simulink model "IIR_Transposed_Direct_Form_II"  (R2012b)
settings: Solver=ode45  StartTime=0.0  StopTime=10.0  RelTol=1e-3
settings Model: Creator=Ahmad  LastModifiedBy=Ahmad

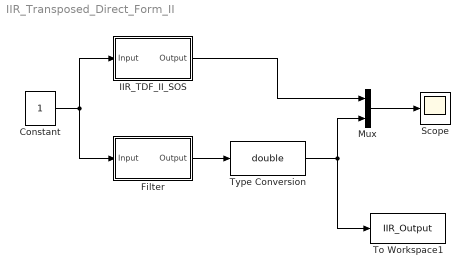
== system IIR_Transposed_Direct_Form_II ==
  Constant : Constant  VectorParams1D=off  OutDataTypeStr=double  SampleTime=1/50e6
  Filter : Subsystem  Tag=FilterWizardSubSystem
      settings: ErrorFcn=dspFilterRealizedInBasicElemsAlgLoopErrFcnCallback
  IIR_TDF_II_SOS : Subsystem  Tag=FilterWizardSubSystem
      settings: ErrorFcn=dspFilterRealizedInBasicElemsAlgLoopErrFcnCallback
  Mux : Mux  Inputs=2
  Scope : Scope
      settings: YMin=0.1  YMax=0.85
  To Workspace1 : ToWorkspace  VariableName=IIR_Output  SampleTime=-1  SaveFormat=Timeseries
  Type Conversion : DataTypeConversion  OutDataTypeStr=double
  wires:
  Constant/1 -> Filter/1(Input), IIR_TDF_II_SOS/1(Input)
  Filter/1(Output) -> Type Conversion/1
  Mux/1 -> Scope/1
  IIR_TDF_II_SOS/1(Output) -> Mux/1
  Type Conversion/1 -> To Workspace1/1, Mux/2

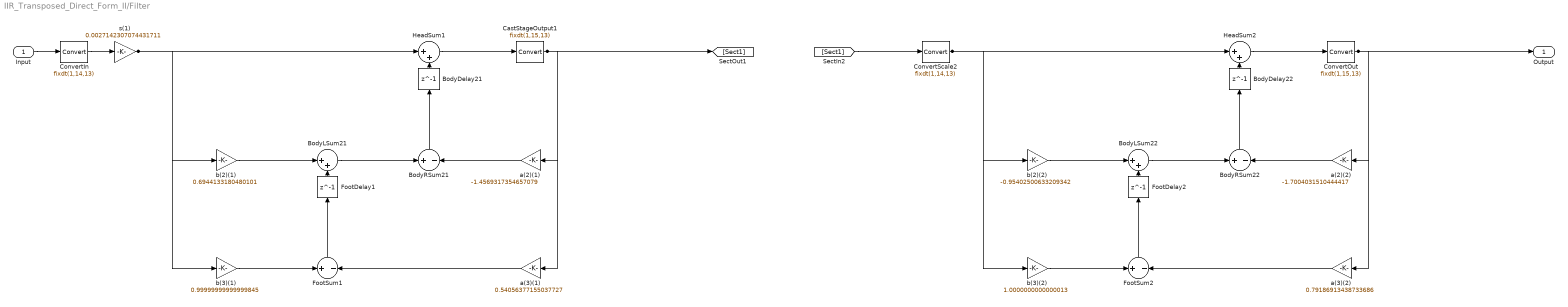
== system IIR_Transposed_Direct_Form_II/Filter ==
  Input : Inport
  BodyDelay21 : Delay  DelayLength=1  InitialCondition=0
  BodyDelay22 : Delay  DelayLength=1  InitialCondition=0
  BodyLSum21 : Sum  Inputs=|++  AccumDataTypeStr=fixdt(1,28,24)  OutDataTypeStr=fixdt(1,28,24)
  BodyLSum22 : Sum  Inputs=|++  AccumDataTypeStr=fixdt(1,28,24)  OutDataTypeStr=fixdt(1,28,24)
  BodyRSum21 : Sum  Inputs=+|-  AccumDataTypeStr=fixdt(1,28,24)  OutDataTypeStr=fixdt(1,28,24)
  BodyRSum22 : Sum  Inputs=+|-  AccumDataTypeStr=fixdt(1,28,24)  OutDataTypeStr=fixdt(1,28,24)
  CastStageOutput1 : DataTypeConversion  OutDataTypeStr=fixdt(1,15,13)
  ConvertIn : DataTypeConversion  OutDataTypeStr=fixdt(1,14,13)  RndMeth=Nearest  SaturateOnIntegerOverflow=on
  ConvertOut : DataTypeConversion  OutDataTypeStr=fixdt(1,15,13)
  ConvertScale2 : DataTypeConversion  OutDataTypeStr=fixdt(1,14,13)
  FootDelay1 : Delay  DelayLength=1  InitialCondition=0
  FootDelay2 : Delay  DelayLength=1  InitialCondition=0
  FootSum1 : Sum  Inputs=+|-  AccumDataTypeStr=fixdt(1,28,24)  OutDataTypeStr=fixdt(1,28,24)
  FootSum2 : Sum  Inputs=+|-  AccumDataTypeStr=fixdt(1,28,24)  OutDataTypeStr=fixdt(1,28,24)
  HeadSum1 : Sum  Inputs=|++  AccumDataTypeStr=fixdt(1,28,24)  OutDataTypeStr=fixdt(1,28,24)
  HeadSum2 : Sum  Inputs=|++  AccumDataTypeStr=fixdt(1,28,24)  OutDataTypeStr=fixdt(1,28,24)
  a(2)(1) : Gain  Gain=-1.4569317354657079  ParamDataTypeStr=fixdt(1,13,11)  OutDataTypeStr=fixdt(1,28,24)
  a(2)(2) : Gain  Gain=-1.7004031510444417  ParamDataTypeStr=fixdt(1,13,11)  OutDataTypeStr=fixdt(1,28,24)
  a(3)(1) : Gain  Gain=0.54056377155037727  ParamDataTypeStr=fixdt(1,13,11)  OutDataTypeStr=fixdt(1,28,24)
  a(3)(2) : Gain  Gain=0.79186913438733686  ParamDataTypeStr=fixdt(1,13,11)  OutDataTypeStr=fixdt(1,28,24)
  b(2)(1) : Gain  Gain=0.6944133180480101  ParamDataTypeStr=fixdt(1,13,11)  OutDataTypeStr=fixdt(1,28,24)
  b(2)(2) : Gain  Gain=-0.95402500633209342  ParamDataTypeStr=fixdt(1,13,11)  OutDataTypeStr=fixdt(1,28,24)
  b(3)(1) : Gain  Gain=0.99999999999999845  ParamDataTypeStr=fixdt(1,13,11)  OutDataTypeStr=fixdt(1,28,24)
  b(3)(2) : Gain  Gain=1.0000000000000013  ParamDataTypeStr=fixdt(1,13,11)  OutDataTypeStr=fixdt(1,28,24)
  s(1) : Gain  Gain=0.0027142307074431711  ParamDataTypeStr=fixdt(1,13,12)  OutDataTypeStr=fixdt(1,14,13)
  Output : Outport
  wires:
  Input/1 -> ConvertIn/1
  s(1)/1 -> HeadSum1/1, b(2)(1)/1, b(3)(1)/1
  HeadSum1/1 -> CastStageOutput1/1
  CastStageOutput1/1 -> [Sect1], a(2)(1)/1, a(3)(1)/1
  b(2)(1)/1 -> BodyLSum21/1
  BodyLSum21/1 -> BodyRSum21/1
  BodyRSum21/1 -> BodyDelay21/1
  a(2)(1)/1 -> BodyRSum21/2
  BodyDelay21/1 -> HeadSum1/2
  b(3)(1)/1 -> FootSum1/1
  FootSum1/1 -> FootDelay1/1
  a(3)(1)/1 -> FootSum1/2
  FootDelay1/1 -> BodyLSum21/2
  ConvertIn/1 -> s(1)/1
  [Sect1] -> ConvertScale2/1
  ConvertScale2/1 -> HeadSum2/1, b(2)(2)/1, b(3)(2)/1
  HeadSum2/1 -> ConvertOut/1
  ConvertOut/1 -> Output/1, a(2)(2)/1, a(3)(2)/1
  b(2)(2)/1 -> BodyLSum22/1
  BodyLSum22/1 -> BodyRSum22/1
  BodyRSum22/1 -> BodyDelay22/1
  a(2)(2)/1 -> BodyRSum22/2
  BodyDelay22/1 -> HeadSum2/2
  b(3)(2)/1 -> FootSum2/1
  FootSum2/1 -> FootDelay2/1
  a(3)(2)/1 -> FootSum2/2
  FootDelay2/1 -> BodyLSum22/2

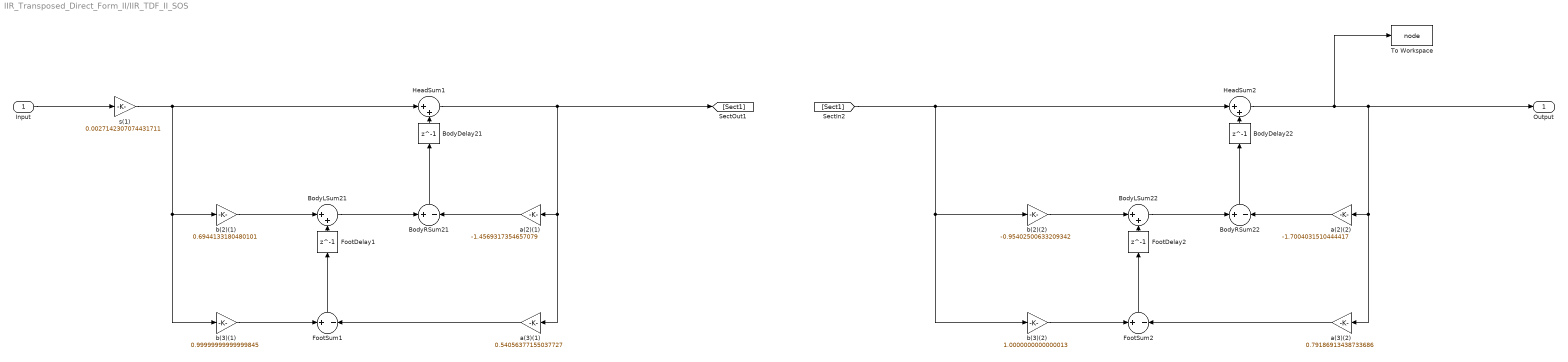
== system IIR_Transposed_Direct_Form_II/IIR_TDF_II_SOS ==
  Input : Inport
  BodyDelay21 : Delay  DelayLength=1  InitialCondition=0
  BodyDelay22 : Delay  DelayLength=1  InitialCondition=0
  BodyLSum21 : Sum  Inputs=|++  RndMeth=Nearest  SaturateOnIntegerOverflow=on  OutDataTypeStr=Inherit: Same as first input
  BodyLSum22 : Sum  Inputs=|++  RndMeth=Nearest  SaturateOnIntegerOverflow=on  OutDataTypeStr=Inherit: Same as first input
  BodyRSum21 : Sum  Inputs=+|-  RndMeth=Nearest  SaturateOnIntegerOverflow=on  OutDataTypeStr=Inherit: Same as first input
  BodyRSum22 : Sum  Inputs=+|-  RndMeth=Nearest  SaturateOnIntegerOverflow=on  OutDataTypeStr=Inherit: Same as first input
  FootDelay1 : Delay  DelayLength=1  InitialCondition=0
  FootDelay2 : Delay  DelayLength=1  InitialCondition=0
  FootSum1 : Sum  Inputs=+|-  RndMeth=Nearest  SaturateOnIntegerOverflow=on  OutDataTypeStr=Inherit: Same as first input
  FootSum2 : Sum  Inputs=+|-  RndMeth=Nearest  SaturateOnIntegerOverflow=on  OutDataTypeStr=Inherit: Same as first input
  HeadSum1 : Sum  Inputs=|++  RndMeth=Nearest  SaturateOnIntegerOverflow=on  OutDataTypeStr=Inherit: Same as first input
  HeadSum2 : Sum  Inputs=|++  RndMeth=Nearest  SaturateOnIntegerOverflow=on  OutDataTypeStr=Inherit: Same as first input
  To Workspace : ToWorkspace  VariableName=node  SampleTime=-1  SaveFormat=Timeseries
  a(2)(1) : Gain  Gain=-1.4569317354657079  ParamDataTypeStr=double  RndMeth=Nearest  SaturateOnIntegerOverflow=on  OutDataTypeStr=Inherit: Same as input
  a(2)(2) : Gain  Gain=-1.7004031510444417  ParamDataTypeStr=double  RndMeth=Nearest  SaturateOnIntegerOverflow=on  OutDataTypeStr=Inherit: Same as input
  a(3)(1) : Gain  Gain=0.54056377155037727  ParamDataTypeStr=double  RndMeth=Nearest  SaturateOnIntegerOverflow=on  OutDataTypeStr=Inherit: Same as input
  a(3)(2) : Gain  Gain=0.79186913438733686  ParamDataTypeStr=double  RndMeth=Nearest  SaturateOnIntegerOverflow=on  OutDataTypeStr=Inherit: Same as input
  b(2)(1) : Gain  Gain=0.6944133180480101  ParamDataTypeStr=double  RndMeth=Nearest  SaturateOnIntegerOverflow=on  OutDataTypeStr=Inherit: Same as input
  b(2)(2) : Gain  Gain=-0.95402500633209342  ParamDataTypeStr=double  RndMeth=Nearest  SaturateOnIntegerOverflow=on  OutDataTypeStr=Inherit: Same as input
  b(3)(1) : Gain  Gain=0.99999999999999845  ParamDataTypeStr=double  RndMeth=Nearest  SaturateOnIntegerOverflow=on  OutDataTypeStr=Inherit: Same as input
  b(3)(2) : Gain  Gain=1.0000000000000013  ParamDataTypeStr=double  RndMeth=Nearest  SaturateOnIntegerOverflow=on  OutDataTypeStr=Inherit: Same as input
  s(1) : Gain  Gain=0.0027142307074431711  ParamDataTypeStr=double  RndMeth=Nearest  SaturateOnIntegerOverflow=on  OutDataTypeStr=Inherit: Same as input
  Output : Outport
  wires:
  Input/1 -> s(1)/1
  s(1)/1 -> b(2)(1)/1, b(3)(1)/1, HeadSum1/1
  HeadSum1/1 -> a(2)(1)/1, a(3)(1)/1, [Sect1]
  b(2)(1)/1 -> BodyLSum21/1
  BodyLSum21/1 -> BodyRSum21/1
  BodyRSum21/1 -> BodyDelay21/1
  a(2)(1)/1 -> BodyRSum21/2
  BodyDelay21/1 -> HeadSum1/2
  b(3)(1)/1 -> FootSum1/1
  FootSum1/1 -> FootDelay1/1
  a(3)(1)/1 -> FootSum1/2
  FootDelay1/1 -> BodyLSum21/2
  [Sect1] -> b(2)(2)/1, b(3)(2)/1, HeadSum2/1
  HeadSum2/1 -> To Workspace/1, a(2)(2)/1, a(3)(2)/1, Output/1
  b(2)(2)/1 -> BodyLSum22/1
  BodyLSum22/1 -> BodyRSum22/1
  BodyRSum22/1 -> BodyDelay22/1
  a(2)(2)/1 -> BodyRSum22/2
  BodyDelay22/1 -> HeadSum2/2
  b(3)(2)/1 -> FootSum2/1
  FootSum2/1 -> FootDelay2/1
  a(3)(2)/1 -> FootSum2/2
  FootDelay2/1 -> BodyLSum22/2
